simulink model "VehicleWithFourSpeedTransmission_Test_R2024a"  (R2025a)
settings: Solver=VariableStepAuto  StartTime=0.0  StopTime=50  RelTol=1e-3
settings Model: Creator=mateu  LastModifiedBy=mateu

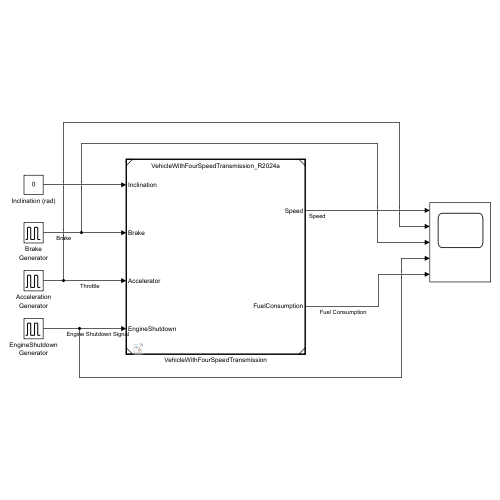
[thumbnail: Simulink's stored preview of the top-level diagram]
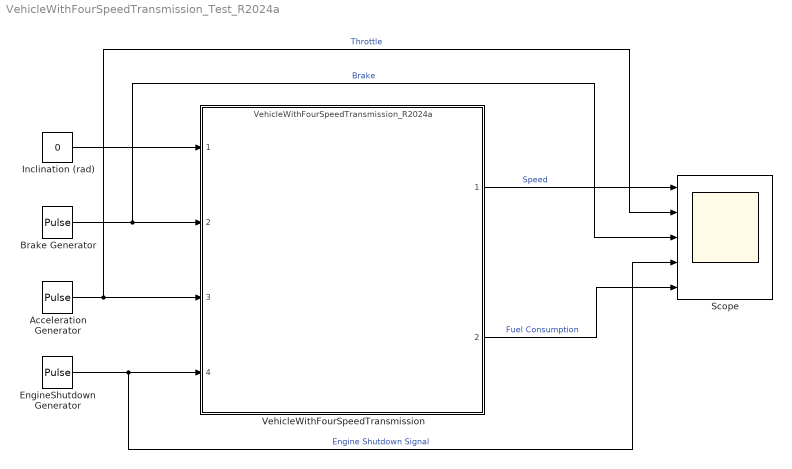
== system VehicleWithFourSpeedTransmission_Test_R2024a ==
  Acceleration Generator : DiscretePulseGenerator  PulseType=Time based  Period=10  PulseWidth=50
  Brake Generator : DiscretePulseGenerator  PulseType=Time based  Period=10  PulseWidth=50  PhaseDelay=5
  EngineShutdown Generator : DiscretePulseGenerator  PulseType=Time based  Period=50  PulseWidth=50  PhaseDelay=25
  Inclination (rad) : Constant  Value=0
  Scope : Scope  NumInputPorts=5
      settings: ActiveDisplayYMinimum=-5.9244  ActiveDisplayYMaximum=100
  VehicleWithFourSpeedTransmission : ModelReference  ModelNameDialog=VehicleWithFourSpeedTransmission_R2024a.slx  SimulationMode=Normal  ModelReferenceVersion=13.15
  wires:
  Acceleration Generator/1 -> Scope/2, VehicleWithFourSpeedTransmission/3  "Throttle"
  Brake Generator/1 -> Scope/3, VehicleWithFourSpeedTransmission/2  "Brake"
  Inclination (rad)/1 -> VehicleWithFourSpeedTransmission/1
  EngineShutdown Generator/1 -> Scope/4, VehicleWithFourSpeedTransmission/4  "Engine Shutdown Signal"
  VehicleWithFourSpeedTransmission/1 -> Scope/1  "Speed"
  VehicleWithFourSpeedTransmission/2 -> Scope/5  "Fuel Consumption"
